simulink model "roz_nieliniowe"  (R2014b)
settings: Solver=ode45  StartTime=0.0  StopTime=Tsym  RelTol=1e-3
undefined symbols (not defined in the file): A, alfa, deltaFc, deltaFd, deltaFh, deltaTc, deltaTd, deltaTh, Fc, Fd, Fh, h0, T0, tau, tauh, Tc, Tciagly, Td, Th, Tskok
settings Model: Creator=Arek  LastModifiedBy=Arek
settings DebuggingCC: SolverPrmCheckMsg=none

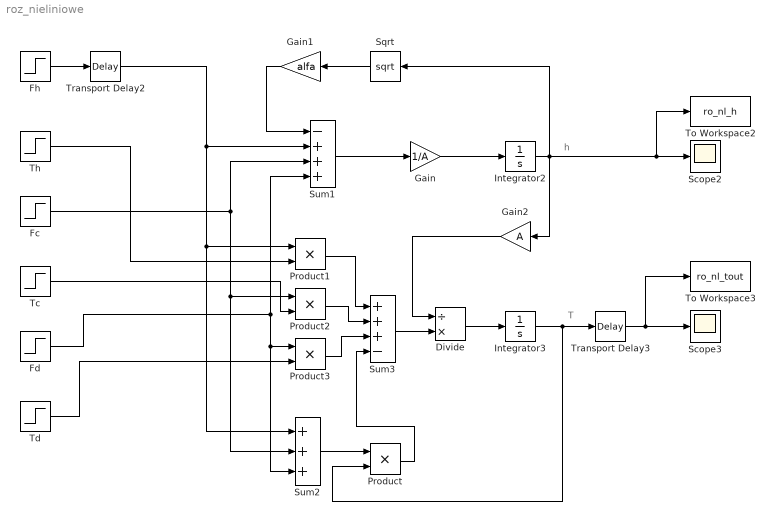
== system roz_nieliniowe ==
  note: T
  note: h
  Divide : Product  Inputs=/*
  Fc : Step  Time=Tskok  Before=Fc  After=Fc+deltaFc  SampleTime=Tciagly
  Fd : Step  Time=Tskok  Before=Fd  After=Fd+deltaFd  SampleTime=Tciagly
  Fh : Step  Time=Tskok  Before=Fh  After=Fh+deltaFh  SampleTime=Tciagly
  Gain : Gain  Gain=1/A
  Gain1 : Gain  Gain=alfa
  Gain2 : Gain  Gain=A
  Integrator2 : Integrator  InitialCondition=h0
  Integrator3 : Integrator  InitialCondition=T0
  Product{,1..3} (4 alike) : Product
  Scope2 : Scope
      settings: SaveName=ScopeData2
  Scope3 : Scope
      settings: SaveName=ScopeData3
  Sqrt : Sqrt  SaturateOnIntegerOverflow=on
  Sum1 : Sum  Inputs=-+++
  Sum2 : Sum  Inputs=+++
  Sum3 : Sum  Inputs=+++-
  Tc : Step  Time=Tskok  Before=Tc  After=Tc+deltaTc  SampleTime=Tciagly
  Td : Step  Time=Tskok  Before=Td  After=Td+deltaTd  SampleTime=Tciagly
  Th : Step  Time=Tskok  Before=Th  After=Th+deltaTh  SampleTime=Tciagly
  To Workspace2 : ToWorkspace  VariableName=ro_nl_h  SaveFormat=Timeseries  SampleTime=-1
  To Workspace3 : ToWorkspace  VariableName=ro_nl_tout  SaveFormat=Timeseries  SampleTime=-1
  Transport Delay2 : TransportDelay  DelayTime=tauh  InitialOutput=Fh
  Transport Delay3 : TransportDelay  DelayTime=tau  InitialOutput=T0
  wires:
  Gain/1 -> Integrator2/1
  Sum1/1 -> Gain/1
  Sqrt/1 -> Gain1/1
  Gain1/1 -> Sum1/1
  Transport Delay2/1 -> Product1/1, Sum2/1, Sum1/2
  Fc/1 -> Sum1/3, Product2/1, Sum2/2
  Fd/1 -> Sum1/4, Product3/1, Sum2/3
  Integrator2/1 -> To Workspace2/1, Scope2/1, Gain2/1, Sqrt/1
  Gain2/1 -> Divide/1
  Divide/1 -> Integrator3/1
  Sum2/1 -> Product/1
  Sum3/1 -> Divide/2
  Product/1 -> Sum3/4
  Product3/1 -> Sum3/3
  Product2/1 -> Sum3/2
  Product1/1 -> Sum3/1
  Td/1 -> Product3/2
  Tc/1 -> Product2/2
  Th/1 -> Product1/2
  Integrator3/1 -> Transport Delay3/1, Product/2
  Transport Delay3/1 -> To Workspace3/1, Scope3/1
  Fh/1 -> Transport Delay2/1
